simulink model "delayMethods"  (R2013a)
settings: Solver=FixedStepDiscrete  StartTime=0.0  StopTime=10.0  FixedStep=0.1  RelTol=1e-3
libraries: simulink x2
settings Model: Creator=User  LastModifiedBy=User

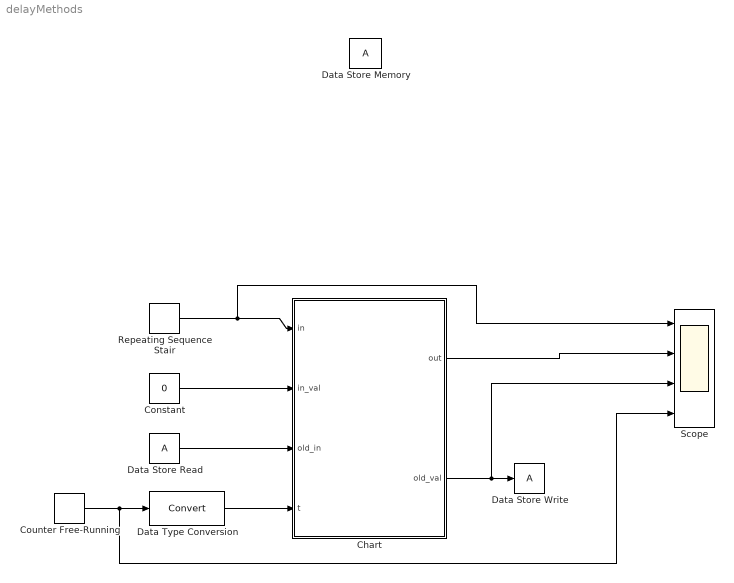
== system delayMethods ==
  Chart : Stateflow chart  TreatAsAtomicUnit=on
  Constant : Constant  Value=0
  Counter Free-Running : simulink/Sources/Counter Free-Running  NumBits=16  tsamp=-1
  Data Store Memory : DataStoreMemory  ReadBeforeWriteMsg=warning  WriteAfterWriteMsg=warning  WriteAfterReadMsg=warning
  Data Store Read : DataStoreRead
  Data Store Write : DataStoreWrite
  Data Type Conversion : DataTypeConversion
  Repeating Sequence Stair : simulink/Sources/Repeating Sequence Stair  OutValues=[3 1 4 2 1].'  tsamp=-1  OutMin=[]  OutMax=[]  OutDataTypeStr=double  OutputDataTypeScalingMode=double  OutDataType=fixdt(0,8)  ConRadixGroup=Best Precision: Vector-wise  OutScaling=2^-12
  Scope : Scope  NumInputPorts=4
      settings: YMin=-5~-5~-5~-5  YMax=5~5~5~5
  wires:
  Chart/2(old_val) -> Scope/3, Data Store Write/1
  Data Store Read/1 -> Chart/3(old_in)
  Constant/1 -> Chart/2(in_val)
  Counter Free-Running/1 -> Scope/4, Data Type Conversion/1
  Repeating Sequence Stair/1 -> Scope/1, Chart/1(in)
  Chart/1(out) -> Scope/2
  Data Type Conversion/1 -> Chart/4(t)

== stateflow chart delayMethods/Chart ==
  (default) -> (junction 3)
  (junction 3) -> (junction 5) [order 2] : [t==0]
  (junction 3) -> (junction 1) [order 1] : {
      | out = old_in;
      | old_val = in;
      | }
  (junction 5) -> (junction 6) : {
      | out = in_val;
      | old_val = in;
      | out = old_in;
      | }
  (junction 6) -> (junction 1)
  data: in input double; in_val input double; old_in input double; t input double; out output double; old_val output double
